simulink model "odefun_toruqe_sim"  (R2021a)
settings: Solver=VariableStepAuto  StartTime=0.0  StopTime=4  RelTol=1e-3
model workspace: external: MATLAB File \\thoth.cecs.pdx.edu\Home01\ik2\Desktop\rotary_pendulum\code\simulate.m (data not in the file)
values from neighbouring files (symbols this model uses):
  K = place(A, B, p)    [simulate.m]
settings Model: Creator=ik2  LastModifiedBy=ik2

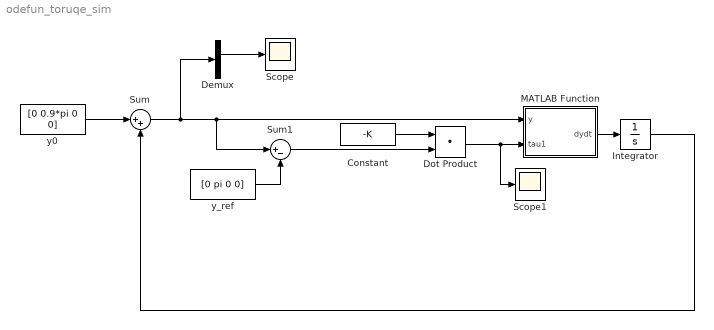
== system odefun_toruqe_sim ==
  Constant : Constant  Value=-K
  Demux : Demux
  Dot Product : DotProduct  InputSameDT=on  OutDataTypeStr=Inherit: Inherit via internal rule
  Integrator : Integrator
  MATLAB Function : MATLAB Function  TreatAsAtomicUnit=on
  Scope : Scope
  Scope1 : Scope
  Sum : Sum  Inputs=|++
  Sum1 : Sum  Inputs=|+-
  y0 : Constant  Value=[0 0.9*pi 0 0]
  y_ref : Constant  Value=[0 pi 0 0]
  wires:
  Integrator/1 -> Sum/2
  y0/1 -> Sum/1
  Sum/1 -> Demux/1, Sum1/1, MATLAB Function/1(y)
  MATLAB Function/1(dydt) -> Integrator/1
  Demux/2 -> Scope/1
  Constant/1 -> Dot Product/1
  y_ref/1 -> Sum1/2
  Sum1/1 -> Dot Product/2
  Dot Product/1 -> Scope1/1, MATLAB Function/2(tau1)

== matlab function odefun_toruqe_sim/MATLAB Function ==
  data: y input; dydt output; tau1 input
function dydt = fcn(y, tau1)

t1 = y(1);
t2 = y(2);
dt1 = y(3);
dt2 = y(4);
tau2 = 0;%0.2*rand() - 0.1; % no disturbance or rand()

ddt1 = f_ddt1(dt1, dt2, t2, tau1, tau2);
ddt2 = f_ddt2(dt1, dt2, t2, tau1, tau2);

dydt = [dt1; dt2; ddt1; ddt2];
